simulink model "modelTest"  (R2023a)
settings: Solver=VariableStepAuto  StartTime=0.0  StopTime=10.0  RelTol=1e-3
settings Model: Creator=Terzo  LastModifiedBy=Terzo

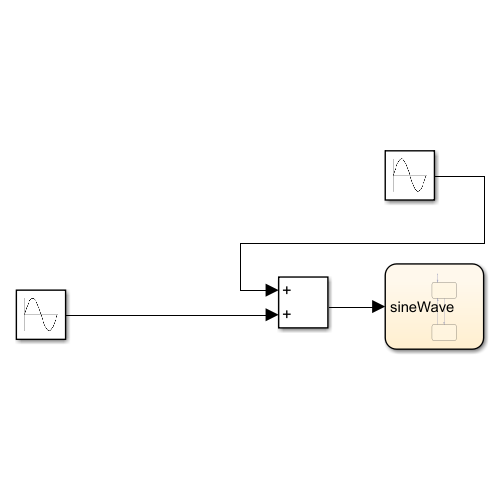
[thumbnail: Simulink's stored preview of the top-level diagram]
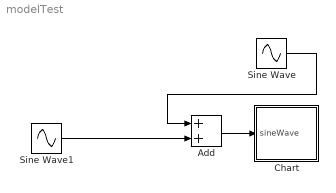
== system modelTest ==
  Add : Sum
  Chart : Stateflow chart  TreatAsAtomicUnit=on
  Sine Wave : Sin  Amplitude=5  Frequency=2  SampleTime=0
  Sine Wave1 : Sin  Frequency=3  SampleTime=0
  wires:
  Sine Wave/1 -> Add/1
  Sine Wave1/1 -> Add/2
  Add/1 -> Chart/1(sineWave)

== stateflow chart modelTest/Chart ==
  state firstState
  state secondState
  (default) -> firstState
  secondState -> firstState : [sineWave > 2]
  firstState -> secondState : [sineWave > 1]
  data: sineWave input; secondV local double; firstV local double
